simulink model "MotorRealDC"  (R2022a)
settings: Solver=VariableStepAuto  StartTime=0.0  StopTime=10.0  RelTol=1e-3
InitFcn:
  | Kt=0.135;
  | Km=0.1534;
  | TL=0;
  | B=0;
  | J=0.0236;
  | L=18e-6;
  | R=0.048;
undefined symbols (not defined in the file): sigbuilder_block
libraries: spsControlledVoltageSourceLib x3, spsCurrentMeasurementLib x2, spsSeriesRLCBranchLib x2, spsDCVoltageSourceLib x1, spsVoltageMeasurementLib x1, spspowerguiLib x1
settings Model: Creator=andre  LastModifiedBy=andre
settings SolverCC: AlgebraicLoopSolver=TrustRegion
settings DebuggingCC: UnconnectedInputMsg=warning  UnconnectedOutputMsg=warning  UnconnectedLineMsg=warning  SFMachineParentedDataDiag=warning

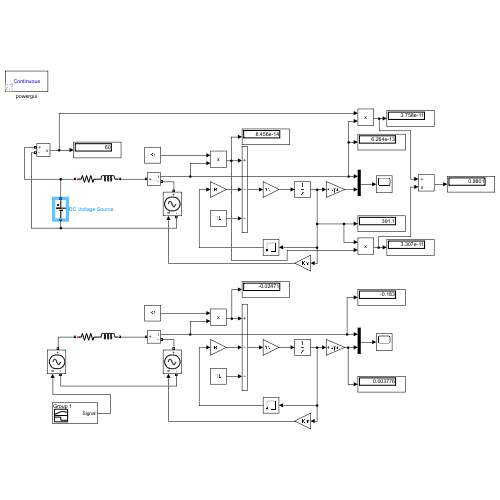
[thumbnail: Simulink's stored preview of the top-level diagram]
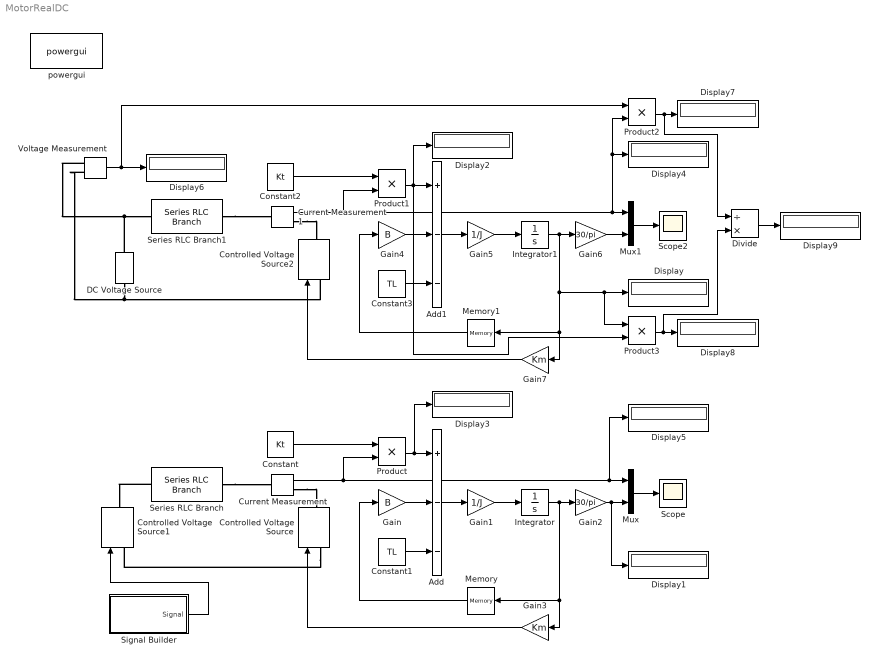
== system MotorRealDC ==
  Add : Sum  Inputs=+--
  Add1 : Sum  Inputs=+--
  Constant : Constant  Value=Kt
  Constant1 : Constant  Value=TL
  Constant2 : Constant  Value=Kt
  Constant3 : Constant  Value=TL
  Controlled Voltage Source : spsControlledVoltageSourceLib/Controlled Voltage Source  Initialize=on  Source_Type=AC  Amplitude=0  Phase=0  Frequency=0  Measurements=None
  Controlled Voltage Source1 : spsControlledVoltageSourceLib/Controlled Voltage Source  Initialize=on  Source_Type=AC  Amplitude=0  Phase=0  Frequency=0  Measurements=None
  Controlled Voltage Source2 : spsControlledVoltageSourceLib/Controlled Voltage Source  Initialize=on  Source_Type=AC  Amplitude=0  Phase=0  Frequency=0  Measurements=None
  Current Measurement : spsCurrentMeasurementLib/Current Measurement  PhasorSimulation=off  OutputType=Complex  PSBequivalent=0
  Current Measurement1 : spsCurrentMeasurementLib/Current Measurement  PhasorSimulation=off  OutputType=Complex  PSBequivalent=0
  DC Voltage Source : spsDCVoltageSourceLib/DC Voltage Source  Amplitude=60  Measurements=None
  Display{,1..9} (10 alike) : Display
  Divide : Product  Inputs=/*
  Gain : Gain  Gain=B
  Gain1 : Gain  Gain=1/J
  Gain2 : Gain  Gain=30/pi
  Gain3 : Gain  Gain=Km
  Gain4 : Gain  Gain=B
  Gain5 : Gain  Gain=1/J
  Gain6 : Gain  Gain=30/pi
  Gain7 : Gain  Gain=Km
  Integrator : Integrator
  Integrator1 : Integrator
  Memory : Memory
  Memory1 : Memory
  Mux : Mux  Inputs=2
  Mux1 : Mux  Inputs=2
  Product{,1..3} (4 alike) : Product
  Scope : Scope
  Scope2 : Scope
  Series RLC Branch : spsSeriesRLCBranchLib/Series RLC Branch  LConnTagsString=__new0  RConnTagsString=__new0  BranchType=RL  Resistance=R  Inductance=L  SetiL0=off  InitialCurrent=0  Capacitance=1e-6  Setx0=off  InitialVoltage=0  Measurements=None
  Series RLC Branch1 : spsSeriesRLCBranchLib/Series RLC Branch  LConnTagsString=__new0  RConnTagsString=__new0  BranchType=RL  Resistance=R  Inductance=L  SetiL0=off  InitialCurrent=0  Capacitance=1e-6  Setx0=off  InitialVoltage=0  Measurements=None
  Signal Builder : Subsystem  Tag=STV Subsys  LoadFcn=sigbuilder_block('load');  StartFcn=sigbuilder_block('start');  StopFcn=sigbuilder_block('stop');  ClipboardFcn=sigbuilder_block('clipboard');  mask(Sigbuilder block){tuvar=[0:10]}
      mask help: Simulink:masks:SigbuilderBlock_MD
      mask init:
      | if ~strcmp(get_param(bdroot(gcbh),'SimulationStatus'),'stopped') tuvar = sigbuilder_block('maskInit'); end
      settings: CopyFcn=sigbuilder_block('copy');  DeleteFcn=sigbuilder_block('delete');  ModelCloseFcn=sigbuilder_block('modelClose');  PreSaveFcn=sigbuilder_block('preSave');  PauseFcn=sigbuilder_block('pause');  ContinueFcn=sigbuilder_block('continue');  NameChangeFcn=sigbuilder_block('namechange');  OpenFcn=sigbuilder_block('open',[5.4 3 1141.2 544.8 ]);  CloseFcn=sigbuilder_block('close');
      mask Display: plot(0, 0, 100, 100,[2, 2, 32, 32, 2], [68, 8, 8, 68, 68],[32, 2], [38, 38], [32, 19, 2],[53, 60, 44], [32, 17, 17, 2],[16, 16, 31, 31]);txt = getActiveGroup(gcbh);text(2, 100, txt,'verticalAlignment', 'top');
  Voltage Measurement : spsVoltageMeasurementLib/Voltage Measurement  PhasorSimulation=off  OutputType=Complex  PSBequivalent=0
  powergui : spspowerguiLib/powergui  Priority=1  SimulationMode=Continuous  SampleTime=50e-6  frequency=60  Iterations=50  frequencyindice=0  Pbase=100e6  ErrMax=1e-4  UnitsV=kV  UnitsW=MW  buscounter=0  FunctionMessages=off  echomessages=off  EnableUseOfTLC=off  CurrentSourceSwitches=off  DisableSnubberDevices=off  DisableRonSwitches=off  DisableVfSwitches=off  DisplayEquations=off  AutomaticDiscreteSolvers=off  SolverType=Tustin/Backward Euler (TBE)  Interpol=off  ExternalGateDelay=off  methode=off  Ts=100  x0status=blocks  SPID=on  SwTol=0  HookPort=off  NonlinearTolerance=1e-4  nMaxIteration=100  ContinueOnMaxIteration=off  RestoreLinks=warning  ResistiveCurrentMeasurement=off  Frange=[0:2:500]  Ylog=off  Xlog=on  ShowGrid=off  save=off  variable=ZData  structure=0  ZoomFFT=off  StartTime=0.0  cycles=1  DisplayStyle=1  fundamental=60  FreqAxis=off  MaxFrequency=1000  frequencyindicesteady=1  RmsSteady=1  display=off
  wires:
  Constant/1 -> Product/1
  Current Measurement/1 -> Product/2, Display5/1, Mux/1
  Gain/1 -> Add/2
  Product/1 -> Display3/1, Add/1
  Constant1/1 -> Add/3
  Add/1 -> Gain1/1
  Gain1/1 -> Integrator/1
  Integrator/1 -> Memory/1, Gain3/1, Gain2/1
  Gain3/1 -> Controlled Voltage Source/1
  Memory/1 -> Gain/1
  Mux/1 -> Scope/1
  Gain2/1 -> Display1/1, Mux/2
  Signal Builder/1(Signal) -> Controlled Voltage Source1/1
  Gain6/1 -> Mux1/2
  Mux1/1 -> Scope2/1
  Memory1/1 -> Gain4/1
  Gain7/1 -> Controlled Voltage Source2/1
  Integrator1/1 -> Gain6/1, Product3/1, Display/1, Gain7/1, Memory1/1
  Gain5/1 -> Integrator1/1
  Add1/1 -> Gain5/1
  Constant3/1 -> Add1/3
  Product1/1 -> Product3/2, Display2/1, Add1/1
  Gain4/1 -> Add1/2
  Current Measurement1/1 -> Product2/2, Display4/1, Mux1/1, Product1/2
  Constant2/1 -> Product1/1
  Voltage Measurement/1 -> Product2/1, Display6/1
  Product2/1 -> Divide/1, Display7/1
  Product3/1 -> Divide/2, Display8/1
  Divide/1 -> Display9/1
  connections:
  Series RLC Branch/LConn1 -- Controlled Voltage Source1/RConn1
  Series RLC Branch/RConn1 -- Current Measurement/LConn1
  Current Measurement/RConn1 -- Controlled Voltage Source/RConn1
  Controlled Voltage Source/LConn1 -- Controlled Voltage Source1/LConn1
  DC Voltage Source/LConn1 -- Voltage Measurement/LConn2 -- Controlled Voltage Source2/LConn1
  Current Measurement1/RConn1 -- Controlled Voltage Source2/RConn1
  Series RLC Branch1/RConn1 -- Current Measurement1/LConn1
  DC Voltage Source/RConn1 -- Voltage Measurement/LConn1 -- Series RLC Branch1/LConn1

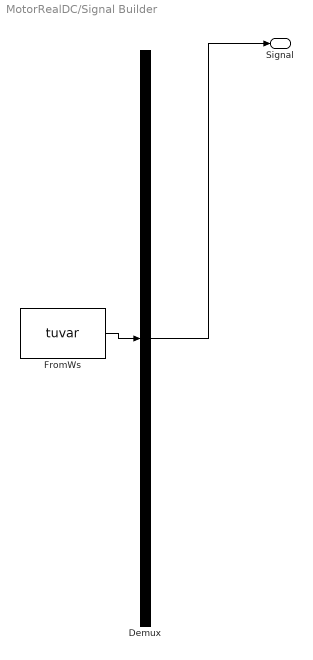
== system MotorRealDC/Signal Builder ==
  Demux : Demux  Tag=STV Demux  Outputs=1
      settings: DisplayOption=none
  FromWs : FromWorkspace  Tag=STV FromWs  VariableName=tuvar
      SigBuilderData=|
      | common.afterFinalStr = 'Extrapolate'
      | common.sampleTime = 0
      | dataSet.timeRange = [0 10]
      | dataSet.name = 'Group 1'
      | sbobj.Groups.Name = 'Group 1'
      | sbobj.Groups.Signals.Name = 'Signal'
      | sbobj.Groups.Signals.XData = [0 2 2 4 4 6 6 8 8 10]
      | sbobj.Groups.Signals.YData = [60 60 30 30 0 0 -60 -60 0 0]
  Signal : Outport  Tag=STV Outport
  wires:
  Demux/1 -> Signal/1
  FromWs/1 -> Demux/1
